simulink subsystem "dsogi"  (R2023a)
settings: Solver=VariableStepAuto  StartTime=0.0  StopTime=10.0  RelTol=1e-3
settings Model: Creator=ASUSTUF  LastModifiedBy=ASUSTUF

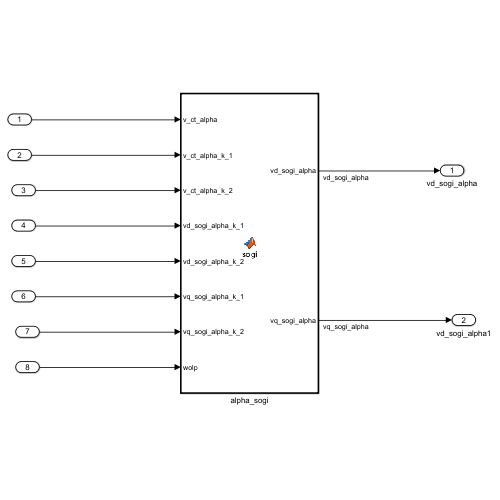
[thumbnail: Simulink's stored preview of the top-level diagram]
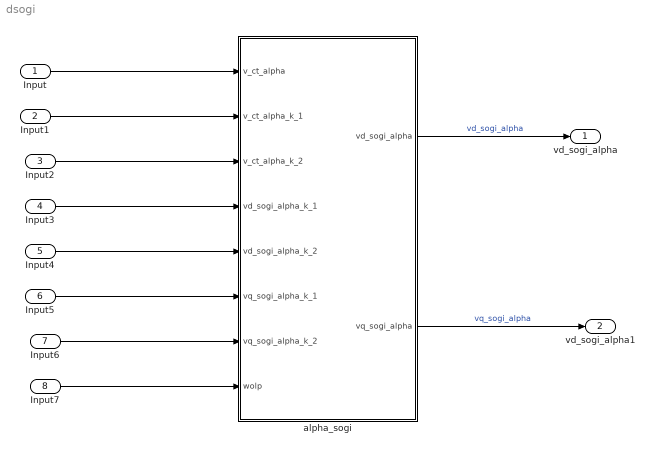
== system dsogi ==
  Input : Inport
  Input1 : Inport  Port=2
  Input2 : Inport  Port=3
  Input3 : Inport  Port=4
  Input4 : Inport  Port=5
  Input5 : Inport  Port=6
  Input6 : Inport  Port=7
  Input7 : Inport  Port=8
  alpha_sogi : MATLAB Function  TreatAsAtomicUnit=on
  vd_sogi_alpha : Outport
  vd_sogi_alpha1 : Outport  Port=2
  wires:
  Input/1 -> alpha_sogi/1(v_ct_alpha)
  Input1/1 -> alpha_sogi/2(v_ct_alpha_k_1)
  Input3/1 -> alpha_sogi/4(vd_sogi_alpha_k_1)
  Input2/1 -> alpha_sogi/3(v_ct_alpha_k_2)
  Input4/1 -> alpha_sogi/5(vd_sogi_alpha_k_2)
  Input6/1 -> alpha_sogi/7(vq_sogi_alpha_k_2)
  Input7/1 -> alpha_sogi/8(wolp)
  Input5/1 -> alpha_sogi/6(vq_sogi_alpha_k_1)
  alpha_sogi/1(vd_sogi_alpha) -> vd_sogi_alpha/1  "vd_sogi_alpha"
  alpha_sogi/2(vq_sogi_alpha) -> vd_sogi_alpha1/1  "vq_sogi_alpha"

== matlab function dsogi/alpha_sogi ==
  data: v_ct_alpha input; vd_sogi_alpha output; v_ct_alpha_k_1 input; v_ct_alpha_k_2 input; vd_sogi_alpha_k_1 input; vd_sogi_alpha_k_2 input; vq_sogi_alpha_k_1 input; vq_sogi_alpha_k_2 input; wolp input; vq_sogi_alpha output
function [vd_sogi_alpha,vq_sogi_alpha]=sogi(v_ct_alpha,v_ct_alpha_k_1,v_ct_alpha_k_2,vd_sogi_alpha_k_1,vd_sogi_alpha_k_2,vq_sogi_alpha_k_1,vq_sogi_alpha_k_2,wolp)

k_sogi1=.5;
wolp=50*2*pi;
fs=10e3;
ts=1/fs;


d_sogi_n1 = (k_sogi1*wolp);
d_sogi_d1 = ((2*fs)-(k_sogi1*wolp)+(ts*.5*wolp*wolp));
d_sogi_d2 = ((ts*wolp*wolp)-(4*fs));
d_sogi_d3 = ((2*fs)+(k_sogi1*wolp)+(ts*.5*wolp*wolp));

vd_sogi_alpha=(( d_sogi_n1*(v_ct_alpha-v_ct_alpha_k_2)-(vd_sogi_alpha_k_1*d_sogi_d2)-(vd_sogi_alpha_k_2*d_sogi_d1) )/d_sogi_d3);

q_sogi_n1=(k_sogi1*wolp*wolp);
q_sogi_n2=(k_sogi1*wolp*wolp*2);
q_sogi_d2=((4*fs*fs)-(2*fs*k_sogi1*wolp)+(wolp*wolp));
q_sogi_d1=((2*wolp*wolp)-(8*fs*fs));
q_sogi_d0=((4*fs*fs)+(2*fs*k_sogi1*wolp)+(wolp*wolp));

vq_sogi_alpha=(((q_sogi_n1*(v_ct_alpha_k_2+v_ct_alpha)+(q_sogi_n2*v_ct_alpha_k_1)) -(vq_sogi_alpha_k_2*q_sogi_d2)-(vq_sogi_alpha_k_1*q_sogi_d1))/q_sogi_d0);



end
